simulink model "ii_90degree"  (R2023b)
settings: Solver=FixedStepDiscrete  StartTime=0.0  StopTime=30  FixedStep=0.01  RelTol=1e-3
undefined symbols (not defined in the file or in its folder): DiscIntNeverNeededParam
libraries: arduinolib x13, simulink x8, mobileRoboticsTrainingLib x1
settings Model: ExtModeTrigDuration=2  Creator=Boitumelo  LastModifiedBy=cameronclark
settings OptimizationCC: EnhancedBackFolding=on  PassReuseOutputArgsAs=Individual arguments  ZeroExternalMemoryAtStartup=off  ZeroInternalMemoryAtStartup=off  MaxStackSize=64  OptimizeBlockOrder=speed  DifferentSizesBufferReuse=on  OptimizationCustomize=off  EfficientTunableParamExpr=on
settings DebuggingCC: ParameterTunabilityLossMsg=error  UnconnectedInputMsg=warning  UnconnectedOutputMsg=warning  UnconnectedLineMsg=warning
settings HardwareCC: ProdBitPerPointer=32  ProdBitPerSizeT=32  ProdBitPerPtrDiffT=32  ProdLargestAtomicInteger=Long  ProdLargestAtomicFloat=Double  ProdWordSize=32  ProdHWDeviceType=ARM Compatible->ARM Cortex  UseEmbeddedCoderFeatures=off  UseSimulinkCoderFeatures=off
settings ModelReferenceCC: EnableRefExpFcnMdlSchedulingChecks=on
settings SFSimCC: MATLABDynamicMemAlloc=off
settings RTWCC: Description=Embedded Coder  SystemTargetFile=ert.tlc  HardwareBoard=Arduino Nano 33 IoT  TemplateMakefile=ert_default_tmf  Toolchain=Arduino ARM  BuildConfiguration=Faster Runs  DLArmComputeVersion=19.05
settings CodeAppCC: ForceParamTrailComments=on  IgnoreCustomStorageClasses=off  OperatorAnnotations=on  SimulinkDataObjDesc=on  SFDataObjDesc=on  InsertBlockDesc=on
settings ERTTargetCC: SupportContinuousTime=on  SupportNonInlinedSFcns=on  SupportVariableSizeSignals=on  ExtModeTransport=3  ExtModeStaticAlloc=on  ExtModeAutomaticAllocSize=off  ExtModeStaticAllocSize=8192  ExtModeMexFile=ext_xcp  ExtModeIntrfLevel=Level2 - Open

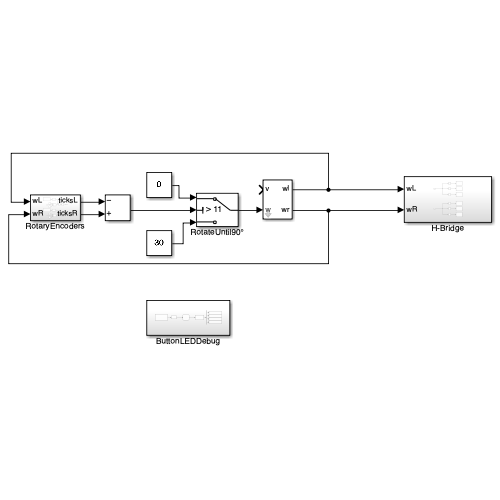
[thumbnail: Simulink's stored preview of the top-level diagram]
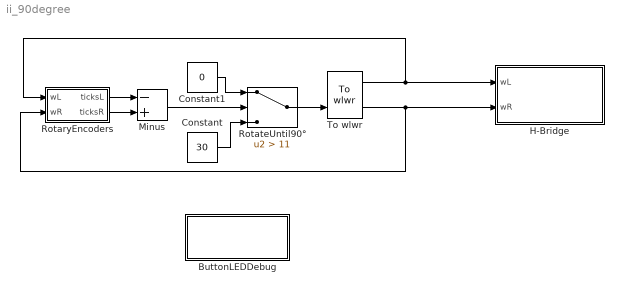
== system ii_90degree ==
  ButtonLEDDebug : Subsystem
  Constant : Constant  Value=30
  Constant1 : Constant  Value=0
  H-Bridge : Subsystem
  Minus : Sum  Inputs=-+
  RotaryEncoders : Subsystem
  RotateUntil90° : Switch  Criteria=u2 > Threshold  Threshold=11  SaturateOnIntegerOverflow=off  InputSameDT=off
  To wlwr : mobileRoboticsTrainingLib/To wlwr  axleLength=0.14  wheelR=0.033
  wires:
  RotateUntil90°/1 -> To wlwr/2
  Constant1/1 -> RotateUntil90°/1
  Minus/1 -> RotateUntil90°/2
  RotaryEncoders/2(ticksR) -> Minus/2
  RotaryEncoders/1(ticksL) -> Minus/1
  To wlwr/1 -> RotaryEncoders/1(wL), H-Bridge/1(wL)
  To wlwr/2 -> RotaryEncoders/2(wR), H-Bridge/2(wR)
  Constant/1 -> RotateUntil90°/3

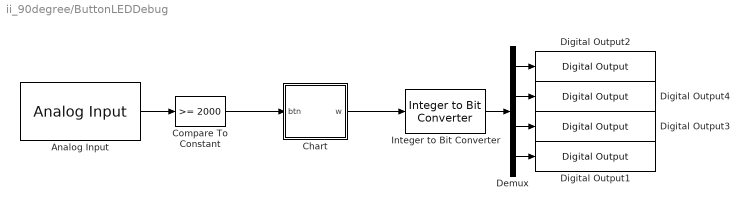
== system ii_90degree/ButtonLEDDebug ==
  Analog Input : arduinolib/Analog Input  pinNumber=0  ReadResultsOnly=off  ConversionTriggerSource=Software  ExternalTriggerType=uint32( 0 )  OutputDataType=uint16  EnableConversionCompleteNotify=off  EnableOuputStatus=off  SampleTime=-1  blockPlatform=arduino
  Chart : Stateflow chart  TreatAsAtomicUnit=on
  Compare To Constant : simulink/Logic and Bit Operations/Compare To Constant  relop=>=  const=2000  OutDataTypeStr=boolean
  Demux : Demux
  Digital Output1 : arduinolib/Digital Output  pinNumber=13  Direction=output  blockPlatform=arduino
  Digital Output2 : arduinolib/Digital Output  pinNumber=8  Direction=output  blockPlatform=arduino
  Digital Output3 : arduinolib/Digital Output  pinNumber=12  Direction=output  blockPlatform=arduino
  Digital Output4 : arduinolib/Digital Output  pinNumber=11  Direction=output  blockPlatform=arduino
  Integer to Bit Converter : simulink/Logic and Bit Operations/Integer to Bit Converter  nbits=4  signedInputValues=Unsigned  bitOrder=MSB first  outDtype=Inherit via internal rule
  wires:
  Chart/1(w) -> Integer to Bit Converter/1
  Demux/2 -> Digital Output4/1
  Demux/1 -> Digital Output2/1
  Demux/4 -> Digital Output1/1
  Demux/3 -> Digital Output3/1
  Analog Input/1 -> Compare To Constant/1
  Integer to Bit Converter/1 -> Demux/1
  Compare To Constant/1 -> Chart/1(btn)

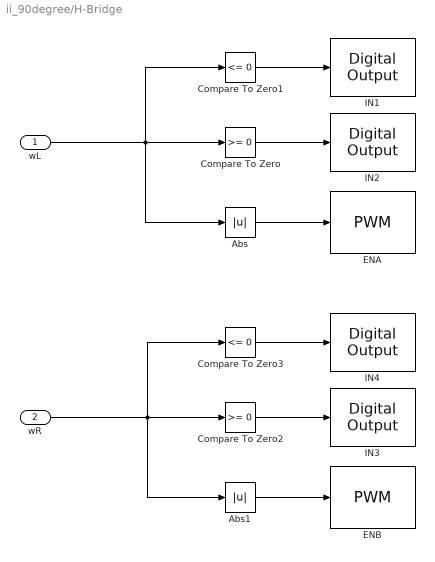
== system ii_90degree/H-Bridge ==
  wL : Inport
  wR : Inport  Port=2
  Abs : Abs  SaturateOnIntegerOverflow=off
  Abs1 : Abs  SaturateOnIntegerOverflow=off
  Compare To Zero : simulink/Logic and Bit Operations/Compare To Zero  relop=>=  OutDataTypeStr=boolean
  Compare To Zero1 : simulink/Logic and Bit Operations/Compare To Zero  relop=<=  OutDataTypeStr=boolean
  Compare To Zero2 : simulink/Logic and Bit Operations/Compare To Zero  relop=>=  OutDataTypeStr=boolean
  Compare To Zero3 : simulink/Logic and Bit Operations/Compare To Zero  relop=<=  OutDataTypeStr=boolean
  ENA : arduinolib/PWM  pinNumber=4  frequencyType=Default  desiredFrequency=490.2  achievableFrequency=490.2
  ENB : arduinolib/PWM  pinNumber=5  frequencyType=Default  desiredFrequency=490.2  achievableFrequency=490.2
  IN1 : arduinolib/Digital Output  pinNumber=2  Direction=output  blockPlatform=arduino
  IN2 : arduinolib/Digital Output  pinNumber=3  Direction=output  blockPlatform=arduino
  IN3 : arduinolib/Digital Output  pinNumber=7  Direction=output  blockPlatform=arduino
  IN4 : arduinolib/Digital Output  pinNumber=6  Direction=output  blockPlatform=arduino
  wires:
  Compare To Zero/1 -> IN2/1
  Compare To Zero1/1 -> IN1/1
  Abs1/1 -> ENB/1
  Compare To Zero2/1 -> IN3/1
  Compare To Zero3/1 -> IN4/1
  wL/1 -> Compare To Zero/1, Abs/1, Compare To Zero1/1
  Abs/1 -> ENA/1
  wR/1 -> Compare To Zero2/1, Compare To Zero3/1, Abs1/1

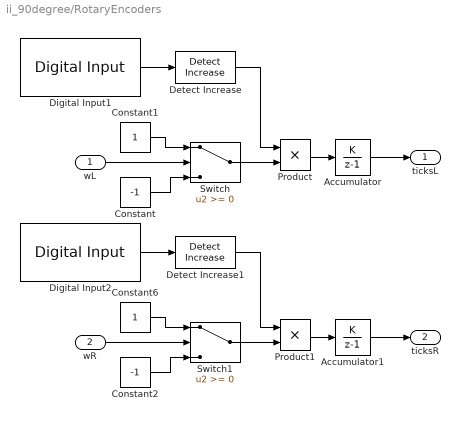
== system ii_90degree/RotaryEncoders ==
  wL : Inport
  wR : Inport  Port=2
  Accumulator : DiscreteIntegrator  IntegratorMethod=Accumulation: Forward Euler  SampleTime=-1  ICPrevOutput=DiscIntNeverNeededParam  ICPrevScaledInput=DiscIntNeverNeededParam
  Accumulator1 : DiscreteIntegrator  IntegratorMethod=Accumulation: Forward Euler  SampleTime=-1  ICPrevOutput=DiscIntNeverNeededParam  ICPrevScaledInput=DiscIntNeverNeededParam
  Constant : Constant  Value=-1
  Constant1 : Constant
  Constant2 : Constant  Value=-1
  Constant6 : Constant
  Detect Increase : simulink/Logic and Bit Operations/Detect Increase  vinit=0.0  OutDataTypeStr=boolean
  Detect Increase1 : simulink/Logic and Bit Operations/Detect Increase  vinit=0.0  OutDataTypeStr=boolean
  Digital Input1 : arduinolib/Digital Input  pinNumber=9  mode=Default  Direction=input  SampleTime=0.1  blockPlatform=arduino
  Digital Input2 : arduinolib/Digital Input  pinNumber=10  mode=Default  Direction=input  SampleTime=0.1  blockPlatform=arduino
  Product : Product
  Product1 : Product
  Switch : Switch  SaturateOnIntegerOverflow=off  InputSameDT=off
  Switch1 : Switch  SaturateOnIntegerOverflow=off  InputSameDT=off
  ticksL : Outport
  ticksR : Outport  Port=2
  wires:
  wL/1 -> Switch/2
  Constant1/1 -> Switch/1
  Constant/1 -> Switch/3
  Digital Input1/1 -> Detect Increase/1
  Switch/1 -> Product/2
  Accumulator/1 -> ticksL/1
  wR/1 -> Switch1/2
  Constant6/1 -> Switch1/1
  Constant2/1 -> Switch1/3
  Accumulator1/1 -> ticksR/1
  Switch1/1 -> Product1/2
  Product/1 -> Accumulator/1
  Detect Increase/1 -> Product/1
  Detect Increase1/1 -> Product1/1
  Digital Input2/1 -> Detect Increase1/1
  Product1/1 -> Accumulator1/1

== stateflow chart ii_90degree/ButtonLEDDebug/Chart ==
  state start
    entry:
    w = 1;
  state out
  state add
    entry:
    w = w + 1;
  (default) -> start
  start -> out
  out -> add : [btn==1]
  add -> out : [btn==0]
  data: w output; btn input
